simulink model "Subsystem"  (R2020b)
settings: Solver=VariableStepAuto  StartTime=0.0  StopTime=10.0  RelTol=1e-3
settings Model: Creator=adity  LastModifiedBy=adity
settings DataIOCC: SaveOutput=off  SaveTime=off

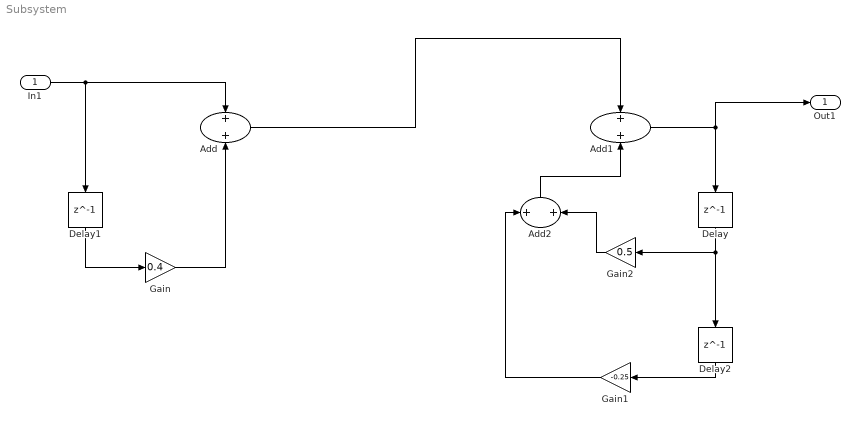
== system Subsystem ==
  In1 : Inport  OutDataTypeStr=double  PortDimensions=1  SampleTime=0
  Add : Sum
  Add1 : Sum
  Add2 : Sum
  Delay : Delay  DelayLength=1
  Delay1 : Delay  DelayLength=1
  Delay2 : Delay  DelayLength=1
  Gain : Gain  Gain=0.4
  Gain1 : Gain  Gain=-0.25
  Gain2 : Gain  Gain=0.5
  Out1 : Outport  OutDataTypeStr=double  PortDimensions=1  SampleTime=0
  wires:
  In1/1 -> Delay1/1, Add/1
  Add1/1 -> Delay/1, Out1/1
  Delay1/1 -> Gain/1
  Add/1 -> Add1/1
  Gain1/1 -> Add2/1
  Delay/1 -> Delay2/1, Gain2/1
  Gain/1 -> Add/2
  Delay2/1 -> Gain1/1
  Gain2/1 -> Add2/2
  Add2/1 -> Add1/2
